simulink model "sysp0 (1)"  (R2024b)
settings: Solver=VariableStepAuto  StartTime=0.0  StopTime=10.0  RelTol=1e-3
libraries: slpidlib x1, simulink x1
settings DataIOCC: ReturnWorkspaceOutputs=off  TimeSaveName=t
settings DebuggingCC: AlgebraicLoopMsg=none  ArtificialAlgebraicLoopMsg=none  MaxConsecutiveZCsMsg=none  OperatingPointInterfaceChecksumMismatchMsg=none

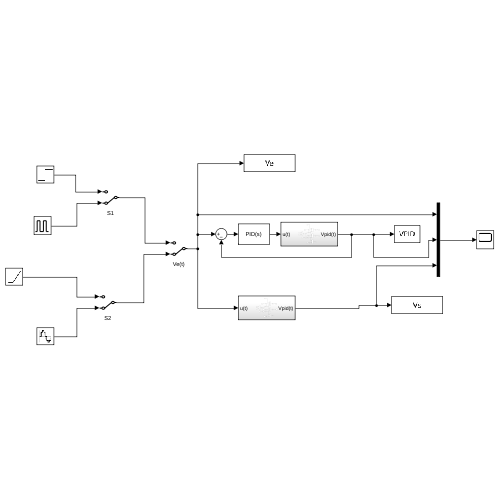
[thumbnail: Simulink's stored preview of the top-level diagram]
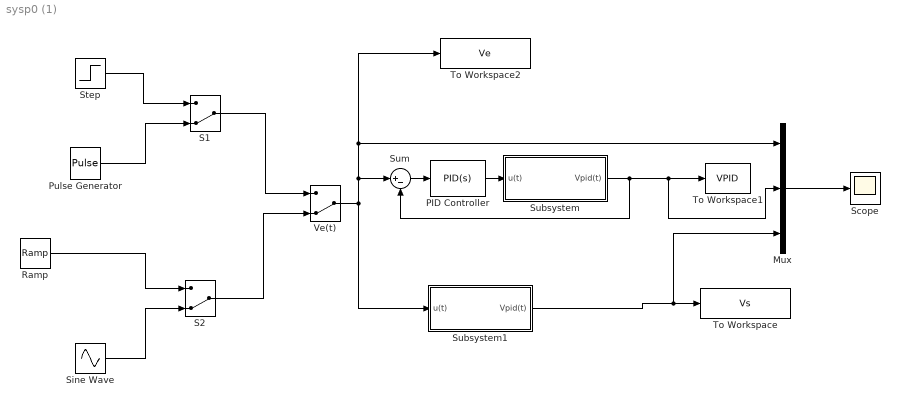
== system sysp0 (1) ==
  Mux : Mux  Inputs=3
  PID Controller : slpidlib/PID Controller  Controller=PID  Form=Parallel  TimeDomain=Continuous-time  UseExternalTs=off  SampleTime=-1  IntegratorMethod=Forward Euler  FilterMethod=Forward Euler  ControllerParametersSource=internal  P=0  I=622.154461673846  UseKiTs=off  D=0  UseExternalDerivativeSource=off  N=100  UseFilter=on  TunerSelectOption=Transfer Function Based (PID Tuner App)  InitialConditionSource=internal  InitialConditionForIntegrator=0  InitialConditionForFilter=0  DifferentiatorICPrevScaledInput=0  ExternalReset=none  TrackingMode=off  Kt=1  LimitOutput=off  SatLimitsSource=internal  UpperSaturationLimit=inf  LowerSaturationLimit=-inf  LinearizeAsGain=on  AntiWindupMode=none  Kb=1  LimitIntegrator=off  UpperIntegratorSaturationLimit=inf  LowerIntegratorSaturationLimit=-inf  POutMin=[]  POutMax=[]  IOutMin=[]  IOutMax=[]  DOutMin=[]  DOutMax=[]  NOutMin=[]  NOutMax=[]  SumOutMin=[]  SumOutMax=[]  SaturationOutMin=[]  SaturationOutMax=[]  PParamMin=[]  PParamMax=[]  IParamMin=[]  IParamMax=[]  DParamMin=[]  DParamMax=[]  NParamMin=[]  NParamMax=[]  KbParamMin=[]  KbParamMax=[]  KtParamMin=[]  KtParamMax=[]  KbOutMin=[]  KbOutMax=[]  KtOutMin=[]  KtOutMax=[]  IntegratorOutMin=[]  IntegratorOutMax=[]  FilterOutMin=[]  FilterOutMax=[]  SumI1OutMin=[]  SumI1OutMax=[]  SumI2OutMin=[]  SumI2OutMax=[]  SumI3OutMin=[]  SumI3OutMax=[]  SumI4OutMin=[]  SumI4OutMax=[]  SumDOutMin=[]  SumDOutMax=[]  DifferentiatorOutMin=[]  DifferentiatorOutMax=[]  FilterDiffOutCoefMin=[]  FilterDiffOutCoefMax=[]  ReciprocalOutMin=[]  ReciprocalOutMax=[]  SumDenOutMin=[]  SumDenOutMax=[]  SumNumOutMin=[]  SumNumOutMax=[]  DivideOutMin=[]  DivideOutMax=[]  UdiffTsProdOutMin=[]  UdiffTsProdOutMax=[]  NTsProdOutMin=[]  NTsProdOutMax=[]  UintegralTsProdOutMin=[]  UintegralTsProdOutMax=[]  UngainTsProdOutMin=[]  UngainTsProdOutMax=[]  ClampingZeroOutDataTypeStr=Inherit: Inherit via back propagation  ClampingZeroOutMin=[]  ClampingZeroOutMax=[]  FilterDenConstantOutDataTypeStr=Inherit: Inherit via back propagation  FilterDenConstantOutMin=[]  FilterDenConstantOutMax=[]  PCopyOutDataTypeStr=Inherit: Inherit via back propagation  PCopyOutMin=[]  PCopyOutMax=[]  NCopyOutDataTypeStr=Inherit: Inherit via back propagation  NCopyOutMin=[]  NCopyOutMax=[]  IntegratorContinuousStateAttributes=''  IntegratorStateMustResolveToSignalObject=off  IntegratorRTWStateStorageClass=Auto  FilterContinuousStateAttributes=''  FilterStateMustResolveToSignalObject=off  FilterRTWStateStorageClass=Auto  ParallelPVariant=InternalParameters  IdealPVariant=Disabled  IVariant=InternalParameters  DVariant=InternalParameters  IntegratorVariant=Continuous  SatVariant=Disabled  AWVariant=Passthrough  PCopyVariant=Disabled  TRVariant=Disabled  FdbkBlocksVariant=Forward  IdealPFdbkVariant=Disabled  SatFdbkVariant=Disabled  DerivativeFilterVariant=ContFilter  NVariant=InternalParameters  NCopyVariant=Disabled  FilterICVariant=InternalICsFilter  IntegratorICVariant=InternalICs  ExternalResetVariant=Disabled  TRSumVariant=Passthrough  SumFdbkVariant=Disabled  SumVariant=Sum_PID  TsampFilterVariant=InternalTs  TsampNgainVariant=Passthrough  TsampIntegralVariant=Disabled_SignalSpec  ExternalSaturationOutDataTypeStr=Inherit: Same as second input  DerivativeSourceVariant=ErrorSignal  PreIntVariant=InternalPreInt
  Pulse Generator : DiscretePulseGenerator  PulseType=Time based  Period=10  PulseWidth=10  PhaseDelay=1
  Ramp : simulink/Sources/Ramp  slope=1/10  start=0  InitialOutput=0
  S1 : ManualSwitch  CurrentSetting=0
  S2 : ManualSwitch  CurrentSetting=0
  Scope : Scope
  Sine Wave : Sin  Frequency=1.5708  SampleTime=0.001
  Step : Step  Time=0  SampleTime=0.001
  Subsystem : Subsystem
  Subsystem1 : Subsystem
  Sum : Sum  Inputs=|+-
  To Workspace : ToWorkspace  VariableName=Vs  SampleTime=-1
  To Workspace1 : ToWorkspace  VariableName=VPID  SampleTime=-1
  To Workspace2 : ToWorkspace  VariableName=Ve  SampleTime=-1
  Ve(t) : ManualSwitch  CurrentSetting=0
  wires:
  Mux/1 -> Scope/1
  Subsystem/1(Vpid(t)) -> To Workspace1/1, Mux/2, Sum/2
  Step/1 -> S1/1
  Pulse Generator/1 -> S1/2
  Sine Wave/1 -> S2/2
  S2/1 -> Ve(t)/2
  S1/1 -> Ve(t)/1
  Ramp/1 -> S2/1
  PID Controller/1 -> Subsystem/1(u(t))
  Sum/1 -> PID Controller/1
  Ve(t)/1 -> Subsystem1/1(u(t)), Sum/1, To Workspace2/1, Mux/1
  Subsystem1/1(Vpid(t)) -> To Workspace/1, Mux/3

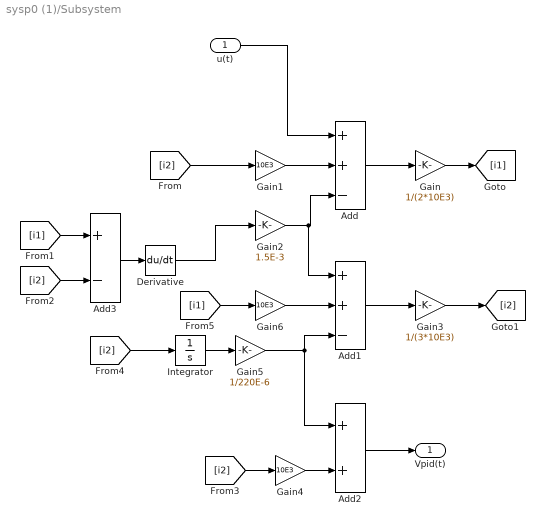
== system sysp0 (1)/Subsystem ==
  u(t) : Inport
  Add : Sum  Inputs=++-
  Add1 : Sum  Inputs=++-
  Add2 : Sum
  Add3 : Sum  Inputs=+-
  Derivative : Derivative
  Gain : Gain  Gain=1/(2*10E3)
  Gain1 : Gain  Gain=10E3
  Gain2 : Gain  Gain=1.5E-3
  Gain3 : Gain  Gain=1/(3*10E3)
  Gain4 : Gain  Gain=10E3
  Gain5 : Gain  Gain=1/220E-6
  Gain6 : Gain  Gain=10E3
  Integrator : Integrator
  Vpid(t) : Outport
  wires:
  u(t)/1 -> Add/1
  Add/1 -> Gain/1
  Gain1/1 -> Add/2
  [i2] -> Gain1/1
  [i1] -> Add3/1
  [i2] -> Add3/2
  Add3/1 -> Derivative/1
  Derivative/1 -> Gain2/1
  Gain2/1 -> Add1/1, Add/3
  Add1/1 -> Gain3/1
  Gain4/1 -> Add2/2
  [i2] -> Gain4/1
  Integrator/1 -> Gain5/1
  Gain5/1 -> Add1/3, Add2/1
  [i2] -> Integrator/1
  Add2/1 -> Vpid(t)/1
  Gain/1 -> [i1]
  Gain3/1 -> [i2]
  Gain6/1 -> Add1/2
  [i1] -> Gain6/1

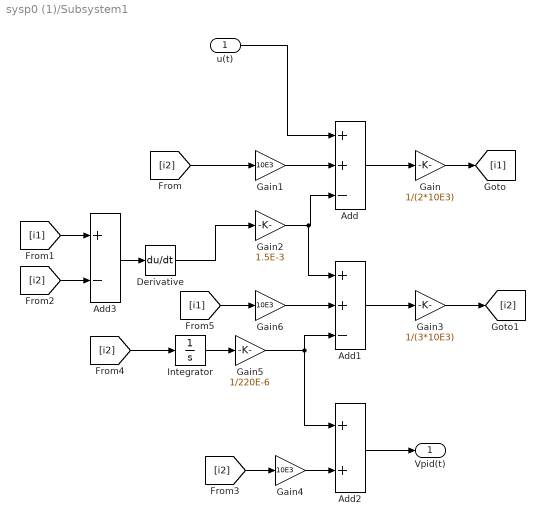
== system sysp0 (1)/Subsystem1 ==
  u(t) : Inport
  Add : Sum  Inputs=++-
  Add1 : Sum  Inputs=++-
  Add2 : Sum
  Add3 : Sum  Inputs=+-
  Derivative : Derivative
  Gain : Gain  Gain=1/(2*10E3)
  Gain1 : Gain  Gain=10E3
  Gain2 : Gain  Gain=1.5E-3
  Gain3 : Gain  Gain=1/(3*10E3)
  Gain4 : Gain  Gain=10E3
  Gain5 : Gain  Gain=1/220E-6
  Gain6 : Gain  Gain=10E3
  Integrator : Integrator
  Vpid(t) : Outport
  wires:
  u(t)/1 -> Add/1
  Add/1 -> Gain/1
  Gain1/1 -> Add/2
  [i2] -> Gain1/1
  [i1] -> Add3/1
  [i2] -> Add3/2
  Add3/1 -> Derivative/1
  Derivative/1 -> Gain2/1
  Gain2/1 -> Add1/1, Add/3
  Add1/1 -> Gain3/1
  Gain4/1 -> Add2/2
  [i2] -> Gain4/1
  Integrator/1 -> Gain5/1
  Gain5/1 -> Add1/3, Add2/1
  [i2] -> Integrator/1
  Add2/1 -> Vpid(t)/1
  Gain/1 -> [i1]
  Gain3/1 -> [i2]
  Gain6/1 -> Add1/2
  [i1] -> Gain6/1
